simulink model "ACAES"  (R2026a)
settings: Solver=ode45  StopTime=t_sim_end  MaxStep=dt  MinStep=1  AbsTol=1e-6
model workspace (MAT data in the model file):
  Constant_mdot_ctrl = 0
  P0 = 101325
  P_comp_rated_W = 100000
  P_turb_rated_W = 100000
  T0 = 293.15
  buy_price = 15
  m_dot_chg_nom = 0.5
  m_dot_dis_nom = 0.6
  sell_price = 10
values from neighbouring files (symbols this model uses):
  cp_air = 1005.0    (= 1005)    [ACAES_params.m]    (also in ACAES_params.mat; CAES_init.m; IDKWHATTHISIS.mat)
  cp_TES = 2000    [ACAES_params.m]    (also in ACAES_params.mat; CAES_init.m = 1900; IDKWHATTHISIS.mat = 1900)
  cv_air = 717.95    [ACAES_params.m]    (also in ACAES_params.mat; CAES_init.m; IDKWHATTHISIS.mat)
  dP_HEX_frac = 0.005    [ACAES_params.m]    (also in ACAES_params.mat; CAES_init.m; IDKWHATTHISIS.mat)
  dt = t_vec(2) - t_vec(1)    [CAES_init.m]    (also in IDKWHATTHISIS.mat = 900)
  epsilon_HEX = 0.92    [ACAES_params.m]    (also in ACAES_params.mat; CAES_init.m = 0.9; IDKWHATTHISIS.mat = 0.9)
  eta_comp_vec = [0.55, 0.68, 0.78, 0.82, 0.82, 0.80, 0.74, 0.66, 0.55]    [CAES_init.m]    (also in IDKWHATTHISIS.mat = [0.55 0.68 0.78 0.82 0.82 0.8 0.74 0.66 0.55])
  eta_gen = 0.97    [ACAES_params.m]    (also in ACAES_params.mat; CAES_extract_results_annual.m = 0.96; CAES_init.m = 0.96; IDKWHATTHISIS.mat = 0.96)
  eta_mech_comp = 0.97    [ACAES_params.m]    (also in ACAES_params.mat; CAES_init.m; IDKWHATTHISIS.mat)
  eta_mech_turb = 0.98    [ACAES_params.m]    (also in ACAES_params.mat; CAES_init.m; IDKWHATTHISIS.mat)
  eta_motor = 0.96    [ACAES_params.m]    (also in ACAES_params.mat; CAES_init.m = 0.95; IDKWHATTHISIS.mat = 0.95)
  eta_turb_vec = [0.65, 0.75, 0.82, 0.85, 0.85, 0.83, 0.79, 0.73, 0.65]    [CAES_init.m]    (also in IDKWHATTHISIS.mat = [0.65 0.75 0.82 0.85 0.85 0.83 0.79 0.73 0.65])
  gamma = 1.4    [ACAES_params.m]    (also in ACAES_params.mat; CAES_init.m; IDKWHATTHISIS.mat)
  Kv_throttle = 0.01    [ACAES_params.m]    (also in ACAES_params.mat; CAES_init.m = 0.005; IDKWHATTHISIS.mat = 0.005)
  leakage_frac = 0.005    [ACAES_params.m]    (also in ACAES_params.mat; CAES_init.m = 0.003; IDKWHATTHISIS.mat = 0.003)
  m_hp_init = P_hp_min*V_hp/(R_air*T0)    (= 47534.8952924)    [ACAES_params.m]    (also in ACAES_params.mat; CAES_init.m = 23767.4476462; IDKWHATTHISIS.mat = 23767.4476462)
  m_TES = 5000    [ACAES_params.m]    (also in ACAES_params.mat; CAES_init.m = 2000; IDKWHATTHISIS.mat = 2000)
  N_stages = 3    [ACAES_params.m]    (also in ACAES_params.mat; CAES_init.m; IDKWHATTHISIS.mat)
  P_hp_init = P_hp_min    (= 4000000)    [ACAES_params.m]    (also in ACAES_params.mat; CAES_init.m; IDKWHATTHISIS.mat)
  P_hp_max = 7e6    (= 7000000)    [ACAES_params.m]    (also in ACAES_params.mat; CAES_init.m; IDKWHATTHISIS.mat)
  P_hp_min = 4e6    (= 4000000)    [ACAES_params.m]    (also in ACAES_params.mat; CAES_init.m; IDKWHATTHISIS.mat)
  P_net_discharge_thresh = 50000    [CAES_init.m]    (also in IDKWHATTHISIS.mat = 5000)
  P_throttle = 4e6    (= 4000000)    [ACAES_params.m]    (also in ACAES_params.mat; CAES_init.m; IDKWHATTHISIS.mat)
  PR_vec = [1.0 1.5 2.0 2.5 3.0 3.5 4.0 4.5 5.0]    [ACAES_params.m]    (also in ACAES_params.mat = [1 1.5 2 2.5 3 3.5 4 4.5 5]; CAES_init.m = [1.0, 1.5, 2.0, 2.5, 3.0, 3.5, 4.0, 4.5, 5.0]; IDKWHATTHISIS.mat = [1 1.5 2 2.5 3 3.5 4 4.5 5])
  R_air = 287.05    [ACAES_params.m]    (also in ACAES_params.mat; CAES_init.m; IDKWHATTHISIS.mat)
  SOC_hp_charge_start = 0.05    [CAES_init.m]    (also in IDKWHATTHISIS.mat)
  SOC_hp_charge_stop = 0.95    [CAES_init.m]    (also in IDKWHATTHISIS.mat)
  SOC_TES_discharge_min = 0.10    (= 0.1)    [CAES_init.m]    (also in IDKWHATTHISIS.mat)
  T_hp_init = T0    (= 293.15)    [ACAES_params.m]    (also in ACAES_params.mat; CAES_init.m; IDKWHATTHISIS.mat)
  T_TES_max = 500    [ACAES_params.m]    (also in ACAES_params.mat; CAES_init.m = 573.15; IDKWHATTHISIS.mat = 573.15)
  tau_valve = 0.5    [ACAES_params.m]    (also in ACAES_params.mat; CAES_init.m = 30; IDKWHATTHISIS.mat = 30)
  UA_TES_wall = 1.5    [CAES_init.m]    (also in IDKWHATTHISIS.mat)
  V_hp = 1000    [ACAES_params.m]    (also in ACAES_params.mat; CAES_init.m = 500; IDKWHATTHISIS.mat = 500)
undefined symbols (not defined in the file or in its folder): DiscIntNeverNeededParam
(part 2 of 2)

== matlab function ACAES/Charging_train/MATLAB Function ==
  data: T_in input; T_out_final output; P_in input; mdot_cmd input; P_hp_current input; T_TES_1 input; T_TES_2 input; T_TES_3 input; enable input; gamma input; cp input; R input; T0 input; eta_comp input; eta_mech input; eta_motor input; epsilon_HEX input; dP_HEX input; leakage input; cp_TES input; m_TES input; PR_vec input; eta_comp_vec input; N_stages input; P_out_final output; mdot_out output; W_dot_elec output; Q_TES_1 output; Q_TES_2 output; Q_TES_3 output; T_TES_1_new output; T_TES_2_new output; T_TES_3_new output; W_dot_loss_comp output; W_dot_loss_HEX output; mdot_leak output
function [T_out_final, P_out_final, mdot_out, W_dot_elec, ...
          Q_TES_1, Q_TES_2, Q_TES_3, T_TES_1_new, T_TES_2_new, T_TES_3_new, ...
          W_dot_loss_comp, W_dot_loss_HEX, mdot_leak] = ...
    compression_physics(T_in, P_in, mdot_cmd, P_hp_current, ...
                        T_TES_1, T_TES_2, T_TES_3, enable, ...
                        gamma, cp, R, T0, eta_comp, eta_mech, eta_motor, ...
                        epsilon_HEX, dP_HEX, leakage, cp_TES, m_TES, ...
                        PR_vec, eta_comp_vec, N_stages)
% COMPRESSION_PHYSICS: 3-stage adiabatic compression with intercooling
% Each stage: compress → cool in HEX → repeat
% Heat from each HEX goes into corresponding TES stage

% Charging fix, hopefully
if ~enable
  % System off
  T_out_final = T_in;
  P_out_final = P_in;
  mdot_out = 0;
  W_dot_elec = 0;

  Q_TES_1 = 0;
  Q_TES_2 = 0;
  Q_TES_3 = 0;

  T_TES_1_new = T_TES_1;
  T_TES_2_new = T_TES_2;
  T_TES_3_new = T_TES_3;

  W_dot_loss_comp = 0;
  W_dot_loss_HEX = 0;
  mdot_leak = 0;
  return;
end

mdot = mdot_cmd;  % requested mass flow [kg/s]

% Safety: avoid division by zero when controller enables charge
% but the commanded mass flow is zero or negative
if mdot <= 1e-6
  T_out_final = T_in;
  P_out_final = P_in;
  mdot_out = 0;
  W_dot_elec = 0;

  Q_TES_1 = 0;
  Q_TES_2 = 0;
  Q_TES_3 = 0;

  T_TES_1_new = T_TES_1;
  T_TES_2_new = T_TES_2;
  T_TES_3_new = T_TES_3;

  W_dot_loss_comp = 0;
  W_dot_loss_HEX = 0;
  mdot_leak = 0;
  return;
end

% Overall pressure ratio per stage (equal stages)
PR_overall = P_hp_current / P_in;     % e.g. 4e6/1e5 = 40
PR_stage   = PR_overall^(1/N_stages); % e.g. 40^(1/3) = 3.42 per stage

% Clamp to physical range
PR_stage = max(1.01, min(PR_stage, PR_vec(end)));

% Off-design isentropic efficiency (same for all stages at same PR_stage)
eta_is = interp1(PR_vec, eta_comp_vec, PR_stage, 'pchip', 'extrap');
eta_is = max(0.40, min(0.92, eta_is));

% Initialize state for stage loop
T_stage = T_in;
P_stage = P_in;
W_dot_comp_total = 0;
W_dot_comp_ideal = 0;
Q_TES = zeros(1, N_stages);
T_TES = [T_TES_1, T_TES_2, T_TES_3];
T_air_stages = zeros(1, N_stages);  % temperature entering each TES stage

for i = 1:N_stages
  % --- COMPRESSION ---
  T_out_is    = T_stage * PR_stage^((gamma-1)/gamma);   % isentropic
  T_out_real  = T_stage + (T_out_is - T_stage) / eta_is; % with loss
  P_out_stage = P_stage * PR_stage;
  
  W_dot_stage_ideal = mdot * cp * (T_out_is - T_stage);    % [W] ideal work
  W_dot_stage_real  = mdot * cp * (T_out_real - T_stage);  % [W] real work
  W_dot_comp_total  = W_dot_comp_total + W_dot_stage_real;
  W_dot_comp_ideal  = W_dot_comp_ideal + W_dot_stage_ideal;
  
  T_air_stages(i) = T_out_real;  % store for HEX calculation
  
  % --- HEAT EXCHANGER (intercooler after each stage) ---
  % HEX transfers heat from hot compressed air to TES fluid
  % HEX effectiveness model: Q = epsilon * C_min * (T_hot_in - T_cold_in)
  C_air  = mdot * cp;
  C_TF   = (mdot * cp / 1900) * 1900;  % balanced flow: m_TF = m_air*(cp_air/cp_TES)
  C_min  = min(C_air, C_TF);
  
  Q_max        = C_min * (T_out_real - T_TES(i));
  Q_HEX        = epsilon_HEX * Q_max;              % [W] actual heat transferred
  Q_TES(i)     = Q_HEX;                            % [W] goes into TES stage i
  
  % Air temperature after HEX (should be near T0 for perfect HEX)
  T_stage = T_out_real - Q_HEX / C_air;
  
  % HEX pressure drop
  P_stage = P_out_stage * (1 - dP_HEX);
end

% Mass leakage (accumulated over all stages)
mdot_leak = leakage * mdot * N_stages;
mdot_out  = mdot - mdot_leak;

% Electrical power (including motor efficiency)
W_dot_elec = W_dot_comp_total / (eta_mech * eta_motor);

% Final outputs
T_out_final = T_stage;    % air temperature entering HP store (should ≈ T0)
P_out_final = P_stage;    % air pressure entering HP store (≈ P_hp_current)

% Losses
W_dot_loss_comp = W_dot_elec - W_dot_comp_ideal;  % [W] compressor + motor loss
W_dot_loss_HEX  = 0;   % HEX losses are captured in TES inefficiency

% New TES temperatures (updated by Q_TES, solved in TES subsystem SS-E)
% We output Q_TES here; TES block integrates to get new T_TES
T_TES_1_new = T_TES_1 + Q_TES(1)/(m_TES*cp_TES) * 1;  % rough estimate, exact in SS-E
T_TES_2_new = T_TES_2 + Q_TES(2)/(m_TES*cp_TES) * 1;
T_TES_3_new = T_TES_3 + Q_TES(3)/(m_TES*cp_TES) * 1;
Q_TES_1 = Q_TES(1); Q_TES_2 = Q_TES(2); Q_TES_3 = Q_TES(3);
end
